simulink model "vehicleModel_23a"  (R2023a)
settings: Solver=VariableStepAuto  StartTime=0.0  StopTime=10.0  RelTol=1e-3
values from neighbouring files (symbols this model uses):
  b1 = b(1,:)    [bicyclekinematicmodel.m]
  b2 = b(2,:)    [bicyclekinematicmodel.m]
undefined symbols (not defined in the file or in its folder): a, linear, position
libraries: ros2lib x8, fuzblock x1
settings Model: Creator=samee  LastModifiedBy=smath24

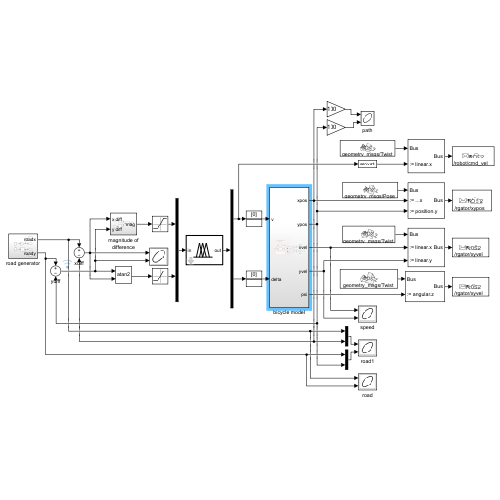
[thumbnail: Simulink's stored preview of the top-level diagram]
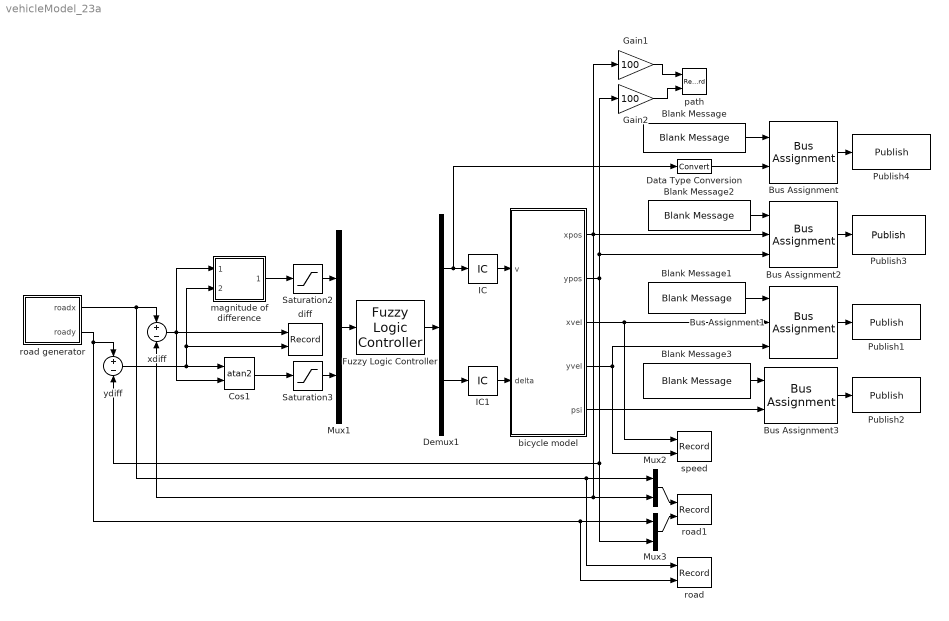
== system vehicleModel_23a ==
  Blank Message : ros2lib/Blank Message  messageClass=Message  entityType=geometry_msgs/Twist  messageType=geometry_msgs/Twist  SampleTime=inf
  Blank Message1 : ros2lib/Blank Message  messageClass=Message  entityType=geometry_msgs/Twist  messageType=geometry_msgs/Twist  SampleTime=inf
  Blank Message2 : ros2lib/Blank Message  messageClass=Message  entityType=geometry_msgs/Pose  messageType=geometry_msgs/Pose  SampleTime=inf
  Blank Message3 : ros2lib/Blank Message  messageClass=Message  entityType=geometry_msgs/Twist  messageType=geometry_msgs/Twist  SampleTime=inf
  Bus Assignment : BusAssignment  AssignedSignals=linear.x
  Bus Assignment1 : BusAssignment  AssignedSignals=linear.x,linear.y
  Bus Assignment2 : BusAssignment  AssignedSignals=position.x,position.y
  Bus Assignment3 : BusAssignment  AssignedSignals=angular.z
  Cos1 : Trigonometry  Operator=atan2
  Data Type Conversion : DataTypeConversion  SaturateOnIntegerOverflow=off  RndMeth=Floor
  Demux1 : Demux  Outputs=2
  Fuzzy Logic Controller : fuzblock/Fuzzy Logic  Controller  FIS=fismatrix  OutputSampleNumber=101  DataType=double  FuzzifiedInputs=off  RuleFiringStrengths=off  RuleOutputs=off  AggregatedOutputs=off  SimulateUsing=Interpreted execution  OutOfRangeInputValueMessage=warning  NoRuleFiredMessage=warning  EmptyOutputFuzzySetMessage=warning
  Gain1 : Gain  Gain=100
  Gain2 : Gain  Gain=100
  IC : InitialCondition  Value=0
  IC1 : InitialCondition  Value=0
  Mux1 : Mux  Inputs=2
  Mux2 : Mux  Inputs=2
  Mux3 : Mux  Inputs=2
  Publish1 : ros2lib/Publish  topicSource=Specify your own  topic=/rgator/xyvel  messageType=geometry_msgs/Twist  QOSHistory=Keep last  QOSDepth=1  QOSReliability=Reliable  QOSDurability=Volatile
  Publish2 : ros2lib/Publish  topicSource=Specify your own  topic=/rgator/xyvel  messageType=geometry_msgs/Twist  QOSHistory=Keep last  QOSDepth=1  QOSReliability=Reliable  QOSDurability=Volatile
  Publish3 : ros2lib/Publish  topicSource=Specify your own  topic=/rgator/xypos  messageType=geometry_msgs/Pose  QOSHistory=Keep last  QOSDepth=1  QOSReliability=Reliable  QOSDurability=Volatile
  Publish4 : ros2lib/Publish  topicSource=Specify your own  topic=/robot/cmd_vel  messageType=geometry_msgs/Twist  QOSHistory=Keep last  QOSDepth=1  QOSReliability=Reliable  QOSDurability=Volatile
  Saturation2 : Saturate  UpperLimit=100  LowerLimit=0  LinearizeAsGain=off
  Saturation3 : Saturate  UpperLimit=1  LowerLimit=-1
  bicycle model : Subsystem
  diff : Record  FileSettingsInternal="{\"entries\":[{\"content\":{\"excelSettings\":{\"content\":{},\"type\":\"Streamout.ExcelSettings\"}},\"type\":\"Streamout.FileSettingStorage\",\"uuid\":\"e11c2646-620e-4821-b31f-06dc8f4cd87f\"}],\"packageUris\":[\"http://schema.mathworks.com/mf0/streamout_blocks/R2020a\"],\"version\":\"1.0\"}"  Layout=[1 1]  SignalsInternal="{\"entries\":[{\"content\":{\"signals\":[{\"content\":{\"blockPath\":[\"vehicleModel_23a/diff\"],\"dimensions\":[1],\"domain\":\"vehicleModel_23a/diff\",\"lineColor\":\"#edb120\",\"plots\":[1],\"port\":1,\"signalID\":48,\"signalName\":\"xdiff\"},\"type\":\"RecordBlkView.Signal\",\"uuid\":\"8016eeb5-851e-4628-929a-2e9a0eab76ef\"},{\"content\":{\"blockPath\":[\"vehicleModel_23a/diff\"],\"dimensions\":[1],\"domain\":\"vehicleModel_23a/diff\",\"lineColor\":\"#7e2f8e\",\"plots\":[1],\"port\":2,\"signalID\":51,\"signalName\":\"ydiff\"},\"type\":\"RecordBlkView.Signal\",\"uuid\":\"cc16506c-ad57-4602-b259-97c109b92ee1\"}]},\"type\":\"RecordBlkView.InputSignals\",\"uuid\":\"c55e6562-a06c-422b-907f-3c73ac4ffa73\"}],\"packageUris\":[\"http://schema.mathworks.com/mf0/streamout_blocks/R2020a\"],\"version\":\"1.0\"}"  VisualizationBindings="{\"xyplotplugin\":{\"info\":[{\"series\":[{\"bindingParametersList\":[{\"parameter\":\"X-Axis\",\"signalID\":48,\"signalName\":\"xdiff\"},{\"parameter\":\"Y-Axis\",\"signalID\":51,\"signalName\":\"ydiff\"}],\"seriesID\":14047}],\"subplotID\":1}]}}"  CompatibilityTag=XY
  magnitude of difference : Subsystem
  path : Record  FileSettingsInternal="{\"entries\":[{\"content\":{\"excelSettings\":{\"content\":{},\"type\":\"Streamout.ExcelSettings\"}},\"type\":\"Streamout.FileSettingStorage\",\"uuid\":\"969ffc95-b704-45a7-aa8e-c06d5542069b\"}],\"packageUris\":[\"http://schema.mathworks.com/mf0/streamout_blocks/R2020a\"],\"version\":\"1.0\"}"  Layout=[1 1]  SignalsInternal="{\"entries\":[{\"content\":{\"signals\":[{\"content\":{\"blockPath\":[\"vehicleModel_23a/path\"],\"dimensions\":[1],\"domain\":\"vehicleModel_23a/path\",\"lineColor\":\"#77ac30\",\"plots\":[1],\"port\":1,\"signalID\":40,\"signalName\":\"Gain\"},\"type\":\"RecordBlkView.Signal\",\"uuid\":\"191c97f3-87f4-45f7-98a3-db8a951101c5\"},{\"content\":{\"blockPath\":[\"vehicleModel_23a/path\"],\"dimensions\":[1],\"domain\":\"vehicleModel_23a/path\",\"lineColor\":\"#4dbeee\",\"plots\":[1],\"port\":2,\"signalID\":43,\"signalName\":\"Gain1\"},\"type\":\"RecordBlkView.Signal\",\"uuid\":\"59408052-173a-49a8-b128-e05ef909a72f\"}]},\"type\":\"RecordBlkView.InputSignals\",\"uuid\":\"c21a6510-29f8-4c3a-bafb-e7d00625e474\"}],\"packageUris\":[\"http://schema.mathworks.com/mf0/streamout_blocks/R2020a\"],\"version\":\"1.0\"}"  VisualizationBindings="{\"xyplotplugin\":{\"info\":[{\"series\":[{\"bindingParametersList\":[{\"parameter\":\"X-Axis\",\"signalID\":40,\"signalName\":\"Gain\"},{\"parameter\":\"Y-Axis\",\"signalID\":43,\"signalName\":\"Gain1\"}],\"seriesID\":43259}],\"subplotID\":1}]}}"  CompatibilityTag=XY
  road : Record  FileSettingsInternal="{\"entries\":[{\"content\":{\"excelSettings\":{\"content\":{},\"type\":\"Streamout.ExcelSettings\"}},\"type\":\"Streamout.FileSettingStorage\",\"uuid\":\"0df6bbcf-3274-4560-95d0-a5963d703d9e\"}],\"packageUris\":[\"http://schema.mathworks.com/mf0/streamout_blocks/R2020a\"],\"version\":\"1.0\"}"  Layout=[1 1]  SignalsInternal="{\"entries\":[{\"content\":{\"signals\":[{\"content\":{\"blockPath\":[\"vehicleModel_23a/road\"],\"dimensions\":[1],\"domain\":\"vehicleModel_23a/road\",\"lineColor\":\"#a2142f\",\"plots\":[1],\"port\":1,\"signalID\":32,\"signalName\":\"road generator:1\"},\"type\":\"RecordBlkView.Signal\",\"uuid\":\"270aa9a5-a50a-4e5f-92ce-1ad2cb7d9aa4\"},{\"content\":{\"blockPath\":[\"vehicleModel_23a/road\"],\"dimensions\":[1],\"domain\":\"vehicleModel_23a/road\",\"lineColor\":\"#139fff\",\"plots\":[1],\"port\":2,\"signalID\":35,\"signalName\":\"road generator:2\"},\"type\":\"RecordBlkView.Signal\",\"uuid\":\"c7f2e2b2-ab32-4e98-a64b-d6370f48c7ec\"}]},\"type\":\"RecordBlkView.InputSignals\",\"uuid\":\"a07b1afe-fa7f-4342-aa7d-6ef05ddddf8b\"}],\"packageUris\":[\"http://schema.mathworks.com/mf0/streamout_blocks/R2020a\"],\"version\":\"1.0\"}"  VisualizationBindings="{\"xyplotplugin\":{\"info\":[{\"series\":[{\"bindingParametersList\":[{\"parameter\":\"X-Axis\",\"signalID\":32,\"signalName\":\"road generator:1\"},{\"parameter\":\"Y-Axis\",\"signalID\":35,\"signalName\":\"road generator:2\"}],\"seriesID\":20322}],\"subplotID\":1}]}}"  CompatibilityTag=XY
  road generator : Subsystem
  road1 : Record  FileSettingsInternal="{\"entries\":[{\"content\":{\"excelSettings\":{\"content\":{},\"type\":\"Streamout.ExcelSettings\"}},\"type\":\"Streamout.FileSettingStorage\",\"uuid\":\"477410f6-626d-4269-8c7e-1abe136939a3\"}],\"packageUris\":[\"http://schema.mathworks.com/mf0/streamout_blocks/R2020a\"],\"version\":\"1.0\"}"  Layout=[1 1]  SignalsInternal="{\"entries\":[{\"content\":{\"signals\":[{\"content\":{\"blockPath\":[\"vehicleModel_23a/road1\"],\"dimensions\":[2],\"domain\":\"vehicleModel_23a/road1\",\"hasChildren\":true,\"lineColor\":\"#a2142f\",\"port\":1,\"signalID\":8,\"signalName\":\"Mux1\"},\"type\":\"RecordBlkView.Signal\",\"uuid\":\"77dfd98c-52af-46ef-b0dc-734aa25e88e8\"},{\"content\":{\"blockPath\":[\"vehicleModel_23a/road1\"],\"channel\":[1],\"dimensions\":[2],\"domain\":\"vehicleModel_23a/road1\",\"lineColor\":\"#139fff\",\"parentID\":8,\"plots\":[1],\"port\":1,\"signalID\":9,\"signalName\":\"Mux1\"},\"type\":\"RecordBlkView.Signal\",\"uuid\":\"676c0de7-8cec-4f7f-b94f-0ccb3ee5a6e9\"},{\"content\":{\"blockPath\":[\"vehicleModel_23a/road1\"],\"channel\":[2],\"dimensions\":[2],\"domain\":\"vehicleModel_23a/road1\",\"lineColor\":\"#fe330a\",\"parentID\":8,\"plots\":[1],\"port\":1,\"signalID\":10,\"signalName\":\"Mux1\"},\"type\":\"RecordBlkView.Signal\",\"uuid\":\"58876b4c-ef76-486f-a2f1-55bbebaf776f\"},{\"content\":{\"blockPath\":[\"vehicleModel_23a/road1\"],\"dimensions\":[2],\"domain\":\"vehicleModel_23a/road1\",\"hasChildren\":true,\"lineColor\":\"#ff6929\",\"port\":2,\"signalID\":15,\"signalName\":\"Mux2\"},\"type\":\"RecordBlkView.Signal\",\"uuid\":\"f8234487-7e31-4a27-aea8-694e6cbc16e5\"},{\"content\":{\"blockPath\":[\"vehicleModel_23a/road1\"],\"channel\":[1],\"dimensions\":[2],\"domain\":\"vehicleModel_23a/road1\",\"lineColor\":\"#b746ff\",\"parentID\":15,\"plots\":[1],\"port\":2,\"signalID\":16,\"signalName\":\"Mux2\"},\"type\":\"RecordBlkView.Signal\",\"uuid\":\"e835b4cc-d614-4dd5-9a5b-e5554e5c85bc\"},{\"content\":{\"blockPath\":[\"vehicleModel_23a/road1\"],\"channel\":[2],\"dimensions\":[2],\"domain\":\"vehicleModel_23a/road1\",\"lineColor\":\"#22b573\",\"parentID\":15,\"plots\":[1],\"port\":2,\"signalID\":17,\"signalName\":\"Mux2\"},\"type\":\"RecordBlkView.Signal\",\"uuid\":\"4f1e4725-4df2-4697-bea0-0df93e51f603\"}]},\"type\":\"RecordBlkView.InputSignals\",\"uuid\":\"de51ccd2-cdc0-4eed-95cf-deac538bd4c0\"}],\"packageUris\":[\"http://schema.mathworks.com/mf0/streamout_blocks/R2020a\"],\"version\":\"1.0\"}"  VisualizationBindings="{\"xyplotplugin\":{\"info\":[{\"series\":[{\"bindingParametersList\":[{\"parameter\":\"X-Axis\",\"signalID\":10,\"signalName\":\"Mux1(2)\"},{\"parameter\":\"Y-Axis\",\"signalID\":16,\"signalName\":\"Mux2(1)\"}],\"seriesID\":13883},{\"bindingParametersList\":[{\"parameter\":\"X-Axis\",\"signalID\":9,\"signalName\":\"Mux1(1)\"},{\"parameter\":\"Y-Axis\",\"signalID\":17,\"signalName\":\"Mux2(2)\"}],\"seriesID\":65135}],\"subplotID\":1}]}}"  CompatibilityTag=XY
  speed : Record  FileSettingsInternal="{\"entries\":[{\"content\":{\"excelSettings\":{\"content\":{},\"type\":\"Streamout.ExcelSettings\"}},\"type\":\"Streamout.FileSettingStorage\",\"uuid\":\"9188d7cb-5000-4f88-9939-3ef4f1a89e9c\"}],\"packageUris\":[\"http://schema.mathworks.com/mf0/streamout_blocks/R2020a\"],\"version\":\"1.0\"}"  Layout=[1 1]  SignalsInternal="{\"entries\":[{\"content\":{\"signals\":[{\"content\":{\"blockPath\":[\"vehicleModel_23a/speed\"],\"dimensions\":[1],\"domain\":\"vehicleModel_23a/speed\",\"lineColor\":\"#ff6929\",\"plots\":[1],\"port\":1,\"signalID\":24,\"signalName\":\"bicycle model:3\"},\"type\":\"RecordBlkView.Signal\",\"uuid\":\"1306c953-2d23-4a8f-88bc-7639a5a32ec7\"},{\"content\":{\"blockPath\":[\"vehicleModel_23a/speed\"],\"dimensions\":[1],\"domain\":\"vehicleModel_23a/speed\",\"lineColor\":\"#b746ff\",\"plots\":[1],\"port\":2,\"signalID\":27,\"signalName\":\"bicycle model:4\"},\"type\":\"RecordBlkView.Signal\",\"uuid\":\"11b28514-ed7b-404a-bef1-14a95db2ac81\"}]},\"type\":\"RecordBlkView.InputSignals\",\"uuid\":\"6efe17d0-8c19-4564-9e27-5a434932449a\"}],\"packageUris\":[\"http://schema.mathworks.com/mf0/streamout_blocks/R2020a\"],\"version\":\"1.0\"}"  VisualizationBindings="{\"xyplotplugin\":{\"info\":[{\"series\":[{\"bindingParametersList\":[{\"parameter\":\"X-Axis\",\"signalID\":24,\"signalName\":\"bicycle model:3\"},{\"parameter\":\"Y-Axis\",\"signalID\":27,\"signalName\":\"bicycle model:4\"}],\"seriesID\":11813}],\"subplotID\":1}]}}"  CompatibilityTag=XY
  xdiff : Sum  Inputs=+-
  ydiff : Sum  Inputs=+-
  wires:
  Mux2/1 -> road1/1
  Saturation2/1 -> Mux1/1
  Fuzzy Logic Controller/1 -> Demux1/1
  Demux1/2 -> IC1/1
  ydiff/1 -> magnitude of difference/2(y diff), diff/2, Cos1/1
  Mux1/1 -> Fuzzy Logic Controller/1
  road generator/2(roady) -> road/2, Mux3/1, ydiff/1
  Blank Message1/1 -> Bus Assignment1/1
  Blank Message/1 -> Bus Assignment/1
  Bus Assignment3/1 -> Publish2/1
  Blank Message3/1 -> Bus Assignment3/1
  Bus Assignment2/1 -> Publish3/1
  road generator/1(roadx) -> xdiff/1, Mux2/1, road/1
  Demux1/1 -> Data Type Conversion/1, IC/1
  Bus Assignment1/1 -> Publish1/1
  bicycle model/5(psi) -> Bus Assignment3/2
  IC1/1 -> bicycle model/2(delta)
  magnitude of difference/1(mag) -> Saturation2/1
  Saturation3/1 -> Mux1/2
  bicycle model/3(xvel) -> speed/1, Bus Assignment1/2
  Gain2/1 -> path/2
  bicycle model/1(xpos) -> Gain1/1, xdiff/2, Mux2/2, Bus Assignment2/2
  Cos1/1 -> Saturation3/1
  xdiff/1 -> Cos1/2, diff/1, magnitude of difference/1(x diff)
  IC/1 -> bicycle model/1(v)
  Mux3/1 -> road1/2
  Gain1/1 -> path/1
  Bus Assignment/1 -> Publish4/1
  bicycle model/4(yvel) -> Bus Assignment1/3, speed/2
  bicycle model/2(ypos) -> Gain2/1, Bus Assignment2/3, Mux3/2, ydiff/2
  Blank Message2/1 -> Bus Assignment2/1
  Data Type Conversion/1 -> Bus Assignment/2

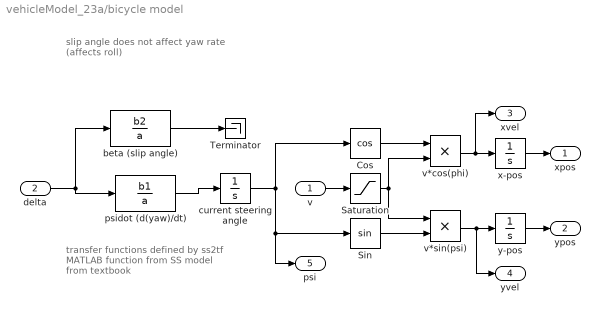
== system vehicleModel_23a/bicycle model ==
  note: transfer functions defined by ss2tf
      | MATLAB function from SS model
      | from textbook
  note: slip angle does not affect yaw rate
      | (affects roll)
  v : Inport
  delta : Inport  Port=2  OutDataTypeStr=double
  Cos : Trigonometry  Operator=cos
  Saturation : Saturate  UpperLimit=30  LowerLimit=-30
  Sin : Trigonometry
  Terminator : Terminator
  beta (slip angle) : TransferFcn  Numerator=b2  Denominator=a  ContinuousStateAttributes='beta'
  current steering angle : Integrator
  psidot (d(yaw)/dt) : TransferFcn  Numerator=b1  Denominator=a  ParameterTunability=Optimized  ContinuousStateAttributes='psidot'
  v*cos(phi) : Product
  v*sin(psi) : Product
  x-pos : Integrator
  y-pos : Integrator
  xpos : Outport
  ypos : Outport  Port=2
  xvel : Outport  Port=3
  yvel : Outport  Port=4
  psi : Outport  Port=5
  wires:
  psidot (d(yaw)/dt)/1 -> current steering angle/1
  v*sin(psi)/1 -> y-pos/1, yvel/1
  current steering angle/1 -> psi/1, Sin/1, Cos/1
  delta/1 -> psidot (d(yaw)/dt)/1, beta (slip angle)/1
  Sin/1 -> v*sin(psi)/2
  v*cos(phi)/1 -> x-pos/1, xvel/1
  Cos/1 -> v*cos(phi)/1
  y-pos/1 -> ypos/1
  x-pos/1 -> xpos/1
  Saturation/1 -> v*cos(phi)/2, v*sin(psi)/1
  v/1 -> Saturation/1
  beta (slip angle)/1 -> Terminator/1

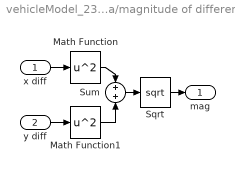
== system vehicleModel_23a/magnitude of difference ==
  x diff : Inport
  y diff : Inport  Port=2
  Math Function : Math  Operator=square
  Math Function1 : Math  Operator=square
  Sqrt : Sqrt
  Sum : Sum  Inputs=+|+
  mag : Outport
  wires:
  Math Function/1 -> Sum/1
  Sum/1 -> Sqrt/1
  Math Function1/1 -> Sum/2
  y diff/1 -> Math Function1/1
  Sqrt/1 -> mag/1
  x diff/1 -> Math Function/1

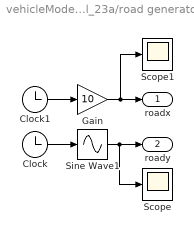
== system vehicleModel_23a/road generator ==
  Clock : Clock
  Clock1 : Clock
  Gain : Gain  Gain=10
  Scope : Scope
  Scope1 : Scope
  Sine Wave1 : Sin  TimeSource=Use external signal  Amplitude=10  Frequency=0.05  Phase=1  SampleTime=0
  roadx : Outport
  roady : Outport  Port=2
  wires:
  Clock/1 -> Sine Wave1/1
  Sine Wave1/1 -> Scope/1, roady/1
  Clock1/1 -> Gain/1
  Gain/1 -> roadx/1, Scope1/1
